simulink model "arm_dynamics_test"  (R2015a)
settings: Solver=ode45  StartTime=0.0  StopTime=10.0  RelTol=1e-3
InitFcn:
  | mdl_aerialmanipulator
  | P = mkgrid(2, 0.1, transl(0,0,1));
  | Tcam = manipulator.fkine([0 3*pi/4 -pi/3 pi/4]);
  | pstar = cam.project(P, 'Tcam', Tcam);
  | 
  | q0 = [0 0 pi/2 0]';
values from neighbouring files (symbols this model uses):
  cam = CentralCamera('focal', 0.0025, 'pixel', 3*1e-6, 'resolution',      [1280 800], 'centre', [640 400], 'name', 'cmucam5')    [mdl_aerialmanipulator.m]
  manipulator = SerialLink([L1 L2 L3 L4], 'name', 'Arm')    [mdl_aerialmanipulator.m]
undefined symbols (not defined in the file or in its folder): aerialmanipulator
libraries: roblocks x10
settings Model: Creator=zhonghang  LastModifiedBy=zhonghang

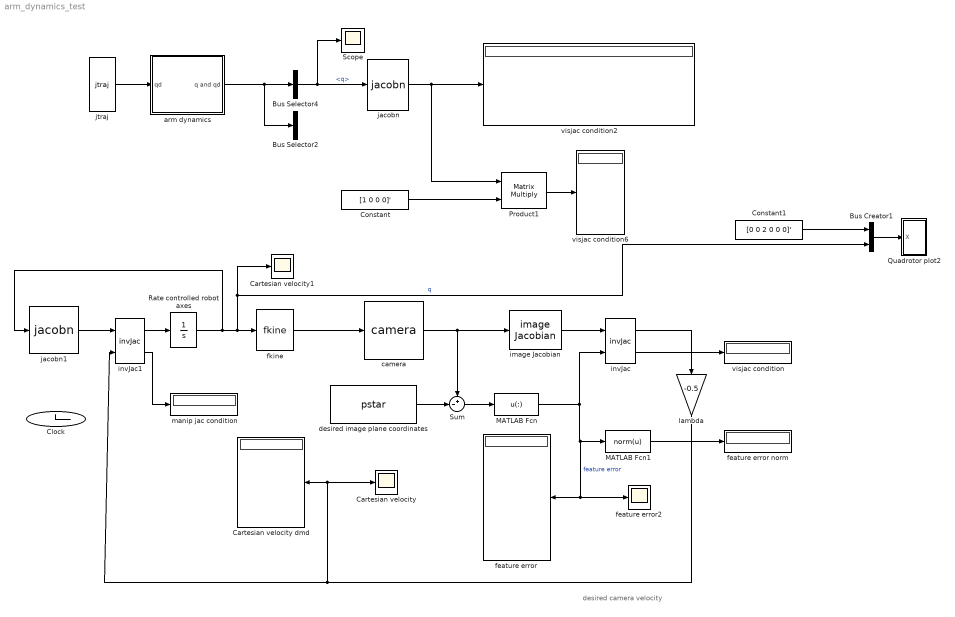
== system arm_dynamics_test ==
  note: desired camera velocity
  Bus Creator1 : BusCreator  Inputs=2
  Bus Selector2 : BusSelector  OutputSignals=qd
  Bus Selector4 : BusSelector  OutputSignals=q
  Cartesian velocity : Scope
      settings: TimeRange=20  YMin=-0.4  YMax=1.9  SaveName=ScopeData2
  Cartesian velocity dmd : Display
      settings: Format=bank
  Cartesian velocity1 : Scope
      settings: TimeRange=10  YMin=-4  YMax=5.5  SaveName=ScopeData3
  Clock : Clock
  Constant : Constant  Value=[1 0 0 0]'
  Constant1 : Constant  Value=[0 0 2 0 0 0]'
  MATLAB Fcn : MATLABFcn  MATLABFcn=u(:)  Output1D=off
  MATLAB Fcn1 : MATLABFcn  MATLABFcn=norm(u)
  Product1 : Product  Multiplication=Matrix(*)
  Quadrotor plot2 : Subsystem  AncestorBlock=roblocks/Robot Graphics/Quadrotor plot  mask{quad=aerialmanipulator, xydim=0.6, zdim=3}
      mask prompts: quad "Model"; xydim "xy-axes dimension"; zdim "z-axis dimension"
      mask help: Animate quadrotor.
      mask Help:
      | This block graphically displays a quadrotor (flying robot).
      | 
      | A new figure is created and A graphical model of a quadrotor is animated
      | to a pose specified by the state vector input to the block.
      | 
      | The state vector is [x y z roll pitch yaw] in world coordinates and the
      | angles are in radians.
      | 
      | Notes:
      | - The dimensions of the vehicle workspace are set by parameters
  Rate controlled robot axes : Integrator  InitialCondition=q0
  Scope : Scope
  Sum : Sum  Inputs=+-|  SaturateOnIntegerOverflow=on  InputSameDT=on  OutDataTypeStr=Inherit: Same as first input
  arm dynamics : Subsystem  mask{robotarm=manipulator, X0=[0 0 0 0]}
      mask prompts: robotarm "robot arm object"; X0 "joint initial value"
  camera : roblocks/Vision/camera  cam=cam  points=P
  desired image plane coordinates : Constant  Value=pstar  VectorParams1D=off
  feature error : Display
      settings: Format=bank
  feature error norm : Display
  feature error2 : Scope
      settings: TimeRange=20  YMin=-150  YMax=150
  fkine : roblocks/Kinematics/fkine  robot=manipulator
  image Jacobian : roblocks/Vision/image Jacobian  cam=cam  z=2
  invJac : roblocks/Vision/invJac
  invJac1 : roblocks/Vision/invJac
  jacobn : roblocks/Kinematics/jacobn  robot=manipulator
  jacobn1 : roblocks/Kinematics/jacobn  robot=manipulator
  jtraj : roblocks/Trajectory/jtraj  q0=[0 0 0 0]  qf=[pi 0 0 0]  tmax=10  ts=-1
  lambda : Gain  Gain=-0.5  SaturateOnIntegerOverflow=on  OutDataTypeStr=Inherit: Same as input  ParamDataTypeStr=Inherit: Same as input
  manip jac condition : Display
  visjac condition : Display
  visjac condition2 : Display
  visjac condition6 : Display
  wires:
  jtraj/2 -> arm dynamics/1(qd)
  arm dynamics/1(q and qd) -> Bus Selector2/1, Bus Selector4/1
  Bus Selector4/1 -> Scope/1, jacobn/1  "<q>"
  jacobn/1 -> visjac condition2/1, Product1/1
  Product1/1 -> visjac condition6/1
  Constant/1 -> Product1/2
  Rate controlled robot axes/1 -> Bus Creator1/2, Cartesian velocity1/1, fkine/1, jacobn1/1  "q"
  jacobn1/1 -> invJac1/1
  invJac1/1 -> Rate controlled robot axes/1
  fkine/1 -> camera/1
  camera/1 -> Sum/1, image Jacobian/1
  Sum/1 -> MATLAB Fcn/1
  desired image plane coordinates/1 -> Sum/2
  MATLAB Fcn/1 -> MATLAB Fcn1/1, feature error2/1, feature error/1, invJac/2  "feature error"
  invJac/2 -> visjac condition/1
  MATLAB Fcn1/1 -> feature error norm/1
  invJac/1 -> lambda/1
  image Jacobian/1 -> invJac/1
  lambda/1 -> Cartesian velocity dmd/1, Cartesian velocity/1, invJac1/2
  invJac1/2 -> manip jac condition/1
  Bus Creator1/1 -> Quadrotor plot2/1(X)
  Constant1/1 -> Bus Creator1/1

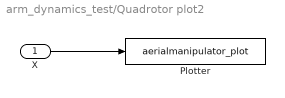
== system arm_dynamics_test/Quadrotor plot2 ==
  X : Inport
  Plotter : S-Function  FunctionName=aerialmanipulator_plot  Parameters=[xydim, zdim], 1, 1,aerialmanipulator
  wires:
  X/1 -> Plotter/1

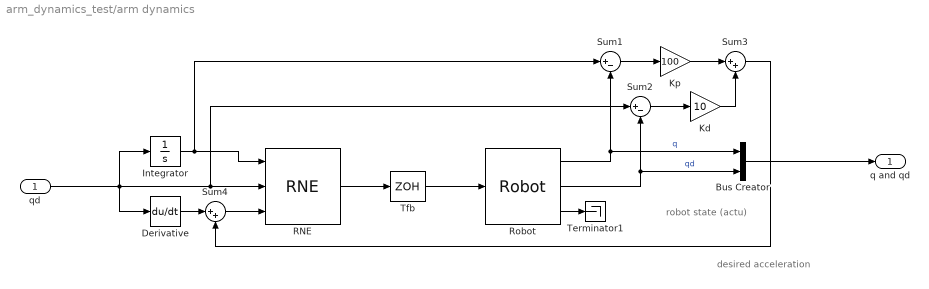
== system arm_dynamics_test/arm dynamics ==
  note: robot state
      | (actu)
  note: desired acceleration
  qd : Inport
  Bus Creator : BusCreator  Inputs=2
  Derivative : Derivative
  Integrator : Integrator
  Kd : Gain  Gain=10  SaturateOnIntegerOverflow=on  OutDataTypeStr=Inherit: Same as input  ParamDataTypeStr=Inherit: Same as input
  Kp : Gain  Gain=100  SaturateOnIntegerOverflow=on  OutDataTypeStr=Inherit: Same as input  ParamDataTypeStr=Inherit: Same as input
  RNE : roblocks/Dynamics/RNE  robot=robotarm  grav=[0 0 9.81]
  Robot : roblocks/Dynamics/Robot  robot=robotarm  q0=X0
  Sum1 : Sum  Inputs=|+-  SaturateOnIntegerOverflow=on  InputSameDT=on  OutDataTypeStr=Inherit: Same as first input
  Sum2 : Sum  Inputs=|+-  SaturateOnIntegerOverflow=on  InputSameDT=on  OutDataTypeStr=Inherit: Same as first input
  Sum3 : Sum  Inputs=|++  SaturateOnIntegerOverflow=on  InputSameDT=on  OutDataTypeStr=Inherit: Same as first input
  Sum4 : Sum  Inputs=|++  SaturateOnIntegerOverflow=on  InputSameDT=on  OutDataTypeStr=Inherit: Same as first input
  Terminator1 : Terminator
  Tfb : ZeroOrderHold  SampleTime=0.01
  q and qd : Outport
  wires:
  Tfb/1 -> Robot/1
  Sum4/1 -> RNE/3
  Robot/2 -> Bus Creator/2, Sum2/2  "qd"
  RNE/1 -> Tfb/1
  Robot/3 -> Terminator1/1
  Sum1/1 -> Kp/1
  Kp/1 -> Sum3/1
  Kd/1 -> Sum3/2
  qd/1 -> Integrator/1, Derivative/1, Sum2/1, RNE/2
  Robot/1 -> Bus Creator/1, Sum1/2  "q"
  Sum2/1 -> Kd/1
  Sum3/1 -> Sum4/2
  Bus Creator/1 -> q and qd/1
  Integrator/1 -> Sum1/1, RNE/1
  Derivative/1 -> Sum4/1
